simulink model "pels25_m"  (Simulink 7.9)
settings: Solver=ode45  StartTime=0.0  StopTime=10.0  RelTol=1e-3
values from neighbouring files (symbols this model uses):
  U = st_Varia('LongNames')    [pels25_i.m]    (also in sofcon_i.m)
  x0 = x0    [pels25_s.m]    (also in sofcon_i.m = []; sofcon_s.m)
undefined symbols (not defined in the file or in its folder): B
settings Model: Creator=M.Sparnaaij  LastModifiedBy=M.Sparnaaij
settings DataIOCC: SignalLoggingName=sigsOut
settings DebuggingCC: SaveWithParameterizedLinksMsg=none  SignalResolutionControl=TryResolveAllWithWarning  SolverPrmCheckMsg=none  MultiTaskDSMMsg=warning  MultiTaskCondExecSysMsg=none  StrictBusMsg=None
settings HardwareCC: TargetUnknown=on
settings RTWCC: IncludeERTFirstTime=on
settings GRTTargetCC: CombineOutputUpdateFcns=off  GRTInterface=on

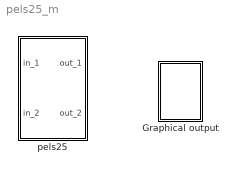
== system pels25_m ==
  Graphical output : Subsystem
      settings: OpenFcn=pels25_g
      mask Display:
      | plot(0,0,100,100,[80,20,20],[20,20,80],[80,69,60,52,45,39,33,28,24,20],[65,65,64,61,57,52,45,37,30,20])
      | disp('');
      | text(100,100,'pels25', 'horizontalAlignment', 'right', 'verticalAlignment', 'top');
  pels25 : Subsystem  Description=pelsof 25
      mask init:
      | filenaam='.\StimelaData\pelsof_p.mat';
      | 
      | [Pn,Fn,Fext]=Fileprop(filenaam);
      | 
      | errstr = st_UniqName(filenaam,'filenaam=''','SubSystem','OpenFcn');
      | if errstr, error([errstr 'The filename "' filenaam '" is already in use. Choose a different filename.']), end
      | 
      | P = pels25_p(filenaam);
      | [B,x0,U]=pels25_i(filenaam);
      settings: OpenFcn=|
      | filenaam='.\StimelaData\pelsof_p.mat';
      | st_ParameterInput('init',gcb,filenaam,'pels25');
      mask Display:
      | image(imread('pels25_f.jpg'))
      | plot(0,0,100,100)
      | disp('')
      | text(50,50,'pels25', 'horizontalAlignment', 'center', 'verticalAlignment', 'middle');
      | text(50,0,Fn, 'horizontalAlignment', 'center', 'verticalAlignment', 'base');

== system pels25_m/Graphical output ==
  note: plotten

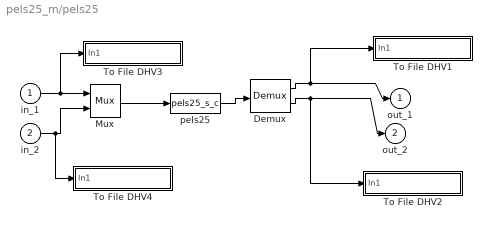
== system pels25_m/pels25 ==
  in_1 : Inport
  in_2 : Inport  Port=2
  Demux : Demux  Outputs=[U.Number B.Measurements]
  Mux : Mux  Inputs=[U.Number B.Setpoints]
  To File DHV1 : Subsystem  mask(To File DHV){naam=[filenaam(1:length(filenaam)-4) '_out.sti']}
      mask prompts: naam "Naam van bestand"
      mask init:
      | set_param([gcb '/To File'],'Filename',naam);
      mask Display: disp(naam)
  To File DHV2 : Subsystem  mask(To File DHV){naam=[filenaam(1:length(filenaam)-4) '_EM.sti']}
      mask prompts: naam "Naam van bestand"
      mask init:
      | set_param([gcb '/To File'],'Filename',naam);
      mask Display: disp(naam)
  To File DHV3 : Subsystem  mask(To File DHV){naam=[filenaam(1:length(filenaam)-4) '_in.sti']}
      mask prompts: naam "Naam van bestand"
      mask init:
      | set_param([gcb '/To File'],'Filename',naam);
      mask Display: disp(naam)
  To File DHV4 : Subsystem  mask(To File DHV){naam=[filenaam(1:length(filenaam)-4) '_ES.sti']}
      mask prompts: naam "Naam van bestand"
      mask init:
      | set_param([gcb '/To File'],'Filename',naam);
      mask Display: disp(naam)
  pels25 : S-Function  FunctionName=pels25_s_c  Parameters=B,x0,U,P  EnableBusSupport=off
  out_1 : Outport  InitialOutput=0
  out_2 : Outport  Port=2  InitialOutput=0
  wires:
  in_2/1 -> To File DHV4/1(In1), Mux/2
  Mux/1 -> pels25/1
  in_1/1 -> To File DHV3/1(In1), Mux/1
  pels25/1 -> Demux/1
  Demux/1 -> To File DHV1/1(In1), out_1/1
  Demux/2 -> To File DHV2/1(In1), out_2/1

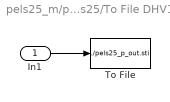
== system pels25_m/pels25/To File DHV1 ==
  In1 : Inport
  To File : ToFile  Filename=./pels25_p_out.sti  MatrixName=pels25out
  wires:
  In1/1 -> To File/1

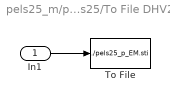
== system pels25_m/pels25/To File DHV2 ==
  In1 : Inport
  To File : ToFile  Filename=./pels25_p_EM.sti  MatrixName=pels25EM
  wires:
  In1/1 -> To File/1

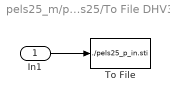
== system pels25_m/pels25/To File DHV3 ==
  In1 : Inport
  To File : ToFile  Filename=./pels25_p_in.sti  MatrixName=pels25in
  wires:
  In1/1 -> To File/1

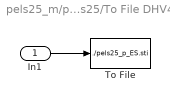
== system pels25_m/pels25/To File DHV4 ==
  In1 : Inport
  To File : ToFile  Filename=./pels25_p_ES.sti  MatrixName=pels25ES
  wires:
  In1/1 -> To File/1
